simulink model "Robot"  (R2019b)
settings: Solver=VariableStepAuto  StartTime=0.0  StopTime=10.0  RelTol=1e-3
undefined symbols (not defined in the file): Tc
settings Model: Creator=manth  LastModifiedBy=manth

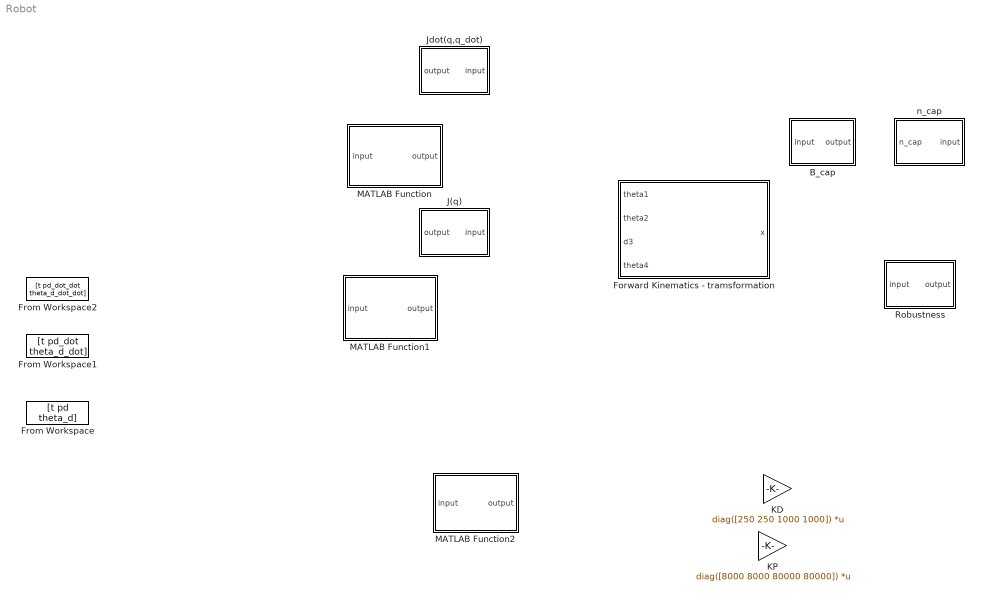
== system Robot ==
  B_cap : MATLAB Function  TreatAsAtomicUnit=on
  Forward Kinematics - tramsformation : MATLAB Function  TreatAsAtomicUnit=on
  From Workspace : FromWorkspace  VariableName=[t pd theta_d]  SampleTime=Tc
  From Workspace1 : FromWorkspace  VariableName=[t pd_dot theta_d_dot]  SampleTime=Tc
  From Workspace2 : FromWorkspace  VariableName=[t pd_dot_dot theta_d_dot_dot]  SampleTime=Tc
  J(q) : MATLAB Function  TreatAsAtomicUnit=on
  Jdot(q,q_dot) : MATLAB Function  TreatAsAtomicUnit=on
  KD : Gain  Gain=diag([250 250 1000 1000])  Multiplication=Matrix(K*u) (u vector)
  KP : Gain  Gain=diag([8000 8000 80000 80000])  Multiplication=Matrix(K*u) (u vector)
  MATLAB Function : MATLAB Function  TreatAsAtomicUnit=on
  MATLAB Function1 : MATLAB Function  TreatAsAtomicUnit=on
  MATLAB Function2 : MATLAB Function  TreatAsAtomicUnit=on
  Robustness : MATLAB Function  TreatAsAtomicUnit=on
  n_cap : MATLAB Function  TreatAsAtomicUnit=on

== matlab function Robot/MATLAB Function ==
  data: input input; output output
function output=Jacobian_inverse(input)
%INPUT is (theta1, theta2, d3, theta4,xd_dot_plus_Ke) 
theta1=input(5,:); d1=0; a1=0.5; alpha1=0; %parameter link1
theta2=input(6,:); d2=0; a2=0.5; alpha2=0; %parameter link2
theta3=0; d3=input(7,:); a3=0; alpha3=0;  %parameter link3
theta4=input(8,:); d4=0; a4=0; alpha4=0;  %parameter link4
 T01=DHmatrix(theta1,d1,a1,alpha1);
 T12=DHmatrix(theta2,d2,a2,alpha2);
 T23=DHmatrix(theta3,d3,a3,alpha3);
 T34=DHmatrix(theta4,d4,a4,alpha4);
 T02=T01*T12;
 T03=T01*T12*T23;
 T04=T01*T12*T23*T34;
P0=[0;0;0];
P1=T01(1:3,4);
P3=T03(1:3,4);
P4=T04(1:3,4);
i
Z0=[0;0;1];
Jv1=cross(Z0,(P4-P0));
Jv2=cross(Z0,(P4-P1));
Jv3=Z0;
Jv4=cross(Z0,(P4-P3));
Jv=[Jv1 Jv2 Jv3 Jv4;1 1 0 1];
output=inv(Jv)*input(1:4,:);
end

function [Mdh] = DHmatrix(theta,d,a,alpha)
%DHMATRIX Summary of this function goes here
%   inputannya DH parameter
Mdh=[cos(theta) -sin(theta)*cos(alpha) sin(theta)*sin(alpha) a*cos(theta);
     sin(theta) cos(theta)*cos(alpha)  -cos(theta)*sin(alpha) a*sin(theta);
     0,sin(alpha),cos(alpha),d;
     0,0,0,1];
end

== matlab function Robot/Forward Kinematics - tramsformation ==
  data: x output; theta1 input; theta2 input; d3 input; theta4 input
function x = forward_kinematics(theta1,theta2,d3,theta4)
     d1=0; a1=0.5; alpha1=0; %parameter link1
     d2=0; a2=0.5; alpha2=0; %parameter link2
theta3=0;  a3=0; alpha3=0;  %parforwardameter link3
     d4=0; a4=0; alpha4=0;  %parameter link4
 T01=DHmatrix(theta1,d1,a1,alpha1);
 T12=DHmatrix(theta2,d2,a2,alpha2);
 T23=DHmatrix(theta3,d3,a3,alpha3);
 T34=DHmatrix(theta4,d4,a4,alpha4);
 T04=T01*T12*T23*T34;
 theta_prime=theta1+theta2+theta4;
x=[T04(1:3,4);theta_prime];
end

function [Mdh] = DHmatrix(theta,d,a,alpha)
%DHMATRIX Summary of this function goes here
%   inputannya DH parameter
Mdh=[cos(theta) -sin(theta)*cos(alpha) sin(theta)*sin(alpha) a*cos(theta);
     sin(theta) cos(theta)*cos(alpha)  -cos(theta)*sin(alpha) a*sin(theta);
     0,sin(alpha),cos(alpha),d;
     0,0,0,1];
end

== matlab function Robot/MATLAB Function1 ==
  data: input input; output output
function output=Jacobian_tranpose(input)
%INPUT is (theta1, theta2, d3, theta4,xd_dot_plus_Ke) 
theta1=input(5,:); d1=0; a1=0.5; alpha1=0; %parameter link1
theta2=input(6,:); d2=0; a2=0.5; alpha2=0; %parameter link2
theta3=0; d3=input(7,:); a3=0; alpha3=0;  %parameter link3
theta4=input(8,:); d4=0; a4=0; alpha4=0;  %parameter link4
 T01=DHmatrix(theta1,d1,a1,alpha1);
 T12=DHmatrix(theta2,d2,a2,alpha2);
 T23=DHmatrix(theta3,d3,a3,alpha3);
 T34=DHmatrix(theta4,d4,a4,alpha4);
 T02=T01*T12;
 T03=T01*T12*T23;
 T04=T01*T12*T23*T34;
P0=[0;0;0];
P1=T01(1:3,4);
P3=T03(1:3,4);
P4=T04(1:3,4);

Z0=[0;0;1];
Jv1=cross(Z0,(P4-P0));
Jv2=cross(Z0,(P4-P1));
Jv3=Z0;
Jv4=cross(Z0,(P4-P3));
Jv=[Jv1 Jv2 Jv3 Jv4;1 1 0 1];
output=Jv'*input(1:4,:);
end

function [Mdh] = DHmatrix(theta,d,a,alpha)
%DHMATRIX Summary of this function goes here
%   inputannya DH parameter
Mdh=[cos(theta) -sin(theta)*cos(alpha) sin(theta)*sin(alpha) a*cos(theta);
     sin(theta) cos(theta)*cos(alpha)  -cos(theta)*sin(alpha) a*sin(theta);
     0,sin(alpha),cos(alpha),d;
     0,0,0,1];
end

== matlab function Robot/Jdot(q,q_dot) ==
  data: input input; output output
function output = Jacobian_dot(input)
% Part 1 Jacobian Differential: J(q)_dot
    theta1 = input(5,:);
    theta2 = input(6,:);
    theta1_dot = input(1,:);
    theta2_dot = input(2,:);
    Jv = [-0.5*(sin(theta1)+sin(theta1+theta2)) -0.5*sin(theta1+theta2) 0 0;
          0.5*(cos(theta1)+cos(theta1+theta2)) 0.5*cos(theta1+theta2) 0 0;
          0 0 -1 0;
          1 1 0 1;];
     Jd = [-0.5*(cos(theta1)*theta1_dot+cos(theta1+theta2)*(theta1_dot)) -0.5*cos(theta1+theta2)*(theta2_dot) 0 0;
           -0.5*(sin(theta1)*theta1_dot+sin(theta1+theta2)*(theta1_dot)) -0.5*sin(theta1+theta2)*(theta2_dot) 0 0;
           0 0 0 0;
           0 0 0 0;];
    q_dot = [input(1,:); input(2,:); input(3,:); input(4,:)];
    output = Jd*q_dot;
end

== matlab function Robot/J(q) ==
  data: input input; output output
function output = Jacobian(input)
% Part 1 Jacobian: J(q)
    theta1 = input(5,:);
    theta2 = input(6,:);
    Jv = [-0.5*(sin(theta1)+sin(theta1+theta2)) -0.5*sin(theta1+theta2) 0 0; 0.5*(cos(theta1)+cos(theta1+theta2)) 0.5*cos(theta1+theta2) 0 0; 0 0 -1 0; 1 1 0 1;];
    q_dot = [input(1,:); input(2,:); input(3,:); input(4,:)];
    output = Jv*q_dot;
end

== matlab function Robot/MATLAB Function2 ==
  data: input input; output output
function output=Jacobian_inverse(input)
%INPUT is (theta1, theta2, d3, theta4,xd_dot_plus_Ke) 
theta1=input(5,:); d1=0; a1=0.5; alpha1=0; %parameter link1
theta2=input(6,:); d2=0; a2=0.5; alpha2=0; %parameter link2
theta3=0; d3=input(7,:); a3=0; alpha3=0;  %parameter link3
theta4=input(8,:); d4=0; a4=0; alpha4=0;  %parameter link4
    Jv = [-0.5*(sin(theta1)+sin(theta1+theta2)) -0.5*sin(theta1+theta2) 0 0;
          0.5*(cos(theta1)+cos(theta1+theta2)) 0.5*cos(theta1+theta2) 0 0;
          0 0 -1 0; 
          1 1 0 1;];
    output = inv(Jv)*input(1:4,:);
end

== matlab function Robot/B_cap ==
  data: input input; output output
function output  = B_cap(input)
    theta2=input(2,:);
    y1=input(5,:);
    y2=input(6,:);
    y3=input(7,:);    
    y4=input(8,:);
    m_l1 = 25;
    m_l2 = 25;
    m_l3 = 10;
    m_l4 = 0;
    I_l1 = 5;
    I_l2 = 5;
    I_l4 = 1;
    I_m1 = 0.0001;
    I_m2 = 0.0001;
    I_m3 = 0.01;
    I_m4 = 0.005;
    l_1 = 0.25;
    l_2 = 0.25;
    k_r1 = 1;
    k_r2 = 1;
    k_r3 = 50;
    k_r4 = 20;
    g = 9.8;
    b11=l_1^2*m_l1+(0.25+l_2^2+l_2*cos(theta2))*m_l2+(0.5+0.5*cos(theta2))*(m_l3+m_l4)+I_l1+I_l2+I_l4+I_m1*k_r1^2+I_m2+I_m3+I_m4;
    b12=(0.5*l_2*cos(theta2)+l_2^2)*m_l2+(0.25+0.25*cos(theta2))*(m_l3+m_l4)+I_l2+I_l4+I_m2*k_r2++I_m3+I_m4;
    b13=-k_r3*I_m3;
    b14=k_r4*I_m4+I_l4;
    b21=b12;
    b22=l_2^2*m_l2+0.25*(m_l4+m_l3)+I_l2+I_l4+I_m2*k_r2^2+I_m4+I_m3;
    b23=-k_r3*I_m3;
    b24=k_r4*I_m4+I_l4;
    b31=b13;
    b32=b23;
    b33=I_m3*k_r3^2+m_l3+m_l4;
    b34=0;
    b41=b14;
    b42=b24;
    b43=b34;
    b44=I_m4*k_r4^2+I_l4;
    B_cap=[b11 b12 b13 b14; b21 b22 b23 b24; b31 b32 b33 b34; b41 b42 b43 b44];
    output=B_cap*[y1 y2 y3 y4]';
end

== matlab function Robot/Robustness ==
  data: input input; output output
function output  = Robustness(input)
%ROBUSTENESS Summary of this function goes here
%   Detailed explanation goes here
e_1=input(1);
e_2=input(2);
e_3=input(3);
e_4=input(4);
e_1_dot=input(5);
e_2_dot=input(6);
e_3_dot=input(7);
e_4_dot=input(8);
D=[zeros(4,4) eye(4)]';
Q=eye(8);
zita=[e_1 e_2 e_3 e_4 e_1_dot e_2_dot e_3_dot e_4_dot]';
z=D'*Q*zita;
n_z=norm(z,2);
epsilon=0.06;
ro=70;
if n_z>=epsilon
    output=ro*z/n_z;
else
    output=ro*z/epsilon;
end

== matlab function Robot/n_cap ==
  data: input input; n_cap output
function n_cap  = n_cap(input)
    theta2=input(2,:);
    theta1_dot=input(5,:);
    theta2_dot=input(6,:);
    d3_dot=input(7,:);
    theta4_dot=input(8,:);
    m_l2 = 25;
    m_l3 = 10;
    m_l4 = 0;
    l_2 = 0.25;
    k_r1 = 1;
    k_r2 = 1;
    k_r3 = 50;
    k_r4 = 20;
    g = 9.8;
    Fv_1 = 0.0001;
    Fv_2 = 0.0001;
    Fv_3 = 0.01;
    Fv_4 = 0.005;
    C_cap=[(-l_2*m_l2*sin(theta2)-0.5*(m_l4+m_l3)*sin(theta2))/2*theta2_dot (-l_2*m_l2*sin(theta2)-0.5*(m_l4+m_l3)*sin(theta2))/2*(theta1_dot+theta2_dot) 0 0;
    -(-l_2*m_l2*sin(theta2)-0.5*(m_l4+m_l3)*sin(theta2))/2*theta1_dot 0 0 0; 0 0 0 0; 0 0 0 0];
    G = [0; 0; -(m_l3+m_l4)*g; 0];
    F = diag([k_r1^2*Fv_1 k_r2^2*Fv_2 k_r3^2*Fv_3 k_r4^2*Fv_4]);
    n_cap = C_cap*[theta1_dot theta2_dot d3_dot theta4_dot]'+F*[theta1_dot theta2_dot d3_dot theta4_dot]'+G;
end
